simulink model "modeldcmotorwithdamper"  (R2019a)
settings: Solver=VariableStepAuto  StartTime=0.0  StopTime=100  RelTol=1e-3
values from neighbouring files (symbols this model uses):
  D_d = 0.0034    [modelrevfinalparameters.mat]
  D_m = 0.00526687727141    [modelrevfinalparameters.mat]
  GR = 0.0526315789474    [modelrevfinalparameters.mat]
  J_l = 0.0012    [modelrevfinalparameters.mat]
  J_m = 0.0001    [modelrevfinalparameters.mat]
  k_e = 0.0064    [modelrevfinalparameters.mat]
  k_t = 0.0071    [modelrevfinalparameters.mat]
  L_a = 0.00487030359254    [modelrevfinalparameters.mat]
  N_d = 1    [modelrevfinalparameters.mat]
  N_l = 1    [modelrevfinalparameters.mat]
  N_m = 1    [modelrevfinalparameters.mat]
  R_a = 2.4    [modelrevfinalparameters.mat]
settings Model: Creator=Yusuf  LastModifiedBy=Yusuf
settings DataIOCC: ReturnWorkspaceOutputs=off
settings DebuggingCC: ArithmeticOperatorsInVariantConditions=warning
settings SFSimCC: SimUseLocalCustomCode=off
settings RTWCC: RTWUseLocalCustomCode=off

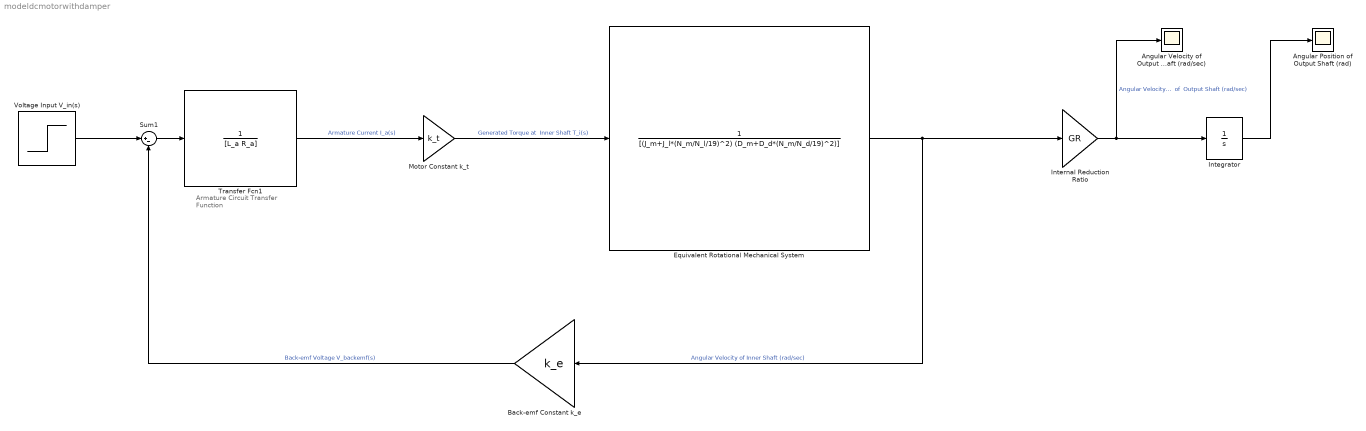
== system modeldcmotorwithdamper ==
  note: Armature Circuit
      | Transfer Function
  Angular Position of Output Shaft (rad) : Scope
  Angular Velocity of Output Shaft (rad/sec) : Scope
  Back-emf Constant k_e : Gain  Gain=k_e
  Equivalent Rotational Mechanical System : TransferFcn  Denominator=[(J_m+J_l*(N_m/N_l/19)^2) (D_m+D_d*(N_m/N_d/19)^2)]
  Integrator : Integrator
  Internal Reduction Ratio : Gain  Gain=GR
  Motor Constant k_t : Gain  Gain=k_t
  Sum1 : Sum  Inputs=|+-
  Transfer Fcn1 : TransferFcn  Denominator=[L_a R_a]
  Voltage Input V_in(s) : Step  Time=0  Before=12  After=12  SampleTime=0
  wires:
  Sum1/1 -> Transfer Fcn1/1
  Equivalent Rotational Mechanical System/1 -> Back-emf Constant k_e/1, Internal Reduction Ratio/1  "Angular Velocity of Inner Shaft (rad/sec)"
  Back-emf Constant k_e/1 -> Sum1/2  "Back-emf Voltage V_backemf(s)"
  Transfer Fcn1/1 -> Motor Constant k_t/1  "Armature Current I_a(s)"
  Motor Constant k_t/1 -> Equivalent Rotational Mechanical System/1  "Generated Torque at  Inner Shaft T_i(s)"
  Integrator/1 -> Angular Position of Output Shaft (rad)/1
  Internal Reduction Ratio/1 -> Angular Velocity of Output Shaft (rad/sec)/1, Integrator/1  "Angular Velocity  of  Output Shaft (rad/sec)"
  Voltage Input V_in(s)/1 -> Sum1/1
